simulink model "Leg_4DOF_HGO_v1"  (R2017a)
settings: Solver=VariableStepAuto  StartTime=0.0  StopTime=10  MaxStep=1e-2  RelTol=1e-3  EnableMultiTasking=on
values from neighbouring files (symbols this model uses):
  Amp = [ 1 ; pi/2*ones(3,1) ]    [Copy_of_Init_4DOF.m]
  Ar = [zeros(4) eye(4); zeros(4) zeros(4)]    [Copy_of_Init_HGO_v2.m]    (also in Init_HGO.m; Init_HGO_v1.m; Init_HGO_zoh_v2.m)
  beta = 10    [Copy_of_Init_4DOF.m]
  BodyContact = [ 4 4 ]    [Copy_of_Init_4DOF.m]
  BodyContactPositions = [ contact_point_h, contact_point_t ]    [Copy_of_Init_4DOF.m]
  Br = [zeros(4); eye(4)]    [Copy_of_Init_HGO_v2.m]    (also in Init_HGO.m; Init_HGO_v1.m; Init_HGO_zoh_v2.m)
  Cr = [eye(4) zeros(4)]    [Copy_of_Init_HGO_v2.m]    (also in Init_HGO.m; Init_HGO_v1.m; Init_HGO_zoh_v2.m)
  dqInit = [ 0 0 0 0 ]'    [Copy_of_Init_4DOF.m]
  G = g*ez    [Copy_of_Init_4DOF.m]
  G_ctrl = g*ez    [Copy_of_Init_4DOF.m]
  h = [ ez -ey -ey -ey ]    [Copy_of_Init_4DOF.m]
  h_ctrl = [ ez -ey -ey -ey ]    [Copy_of_Init_4DOF.m]
  Hmu = [eye(4)/Mu zeros(4); zeros(4) eye(4)/Mu^2]    [Copy_of_Init_HGO_v2.m]    (also in Init_HGO.m; Init_HGO_v1.m; Init_HGO_zoh_v2.m)
  Inertia = [ I_base I_hip I_thigh I_shin I_foot ]    [Copy_of_Init_4DOF.m]
  Inertia_ctrl = [ I_base I_hip I_thigh I_shin I_foot ]    [Copy_of_Init_4DOF.m]
  joint_type = [ 1 0 0 0 ]    [Copy_of_Init_4DOF.m]
  k_b = 10    [Copy_of_Init_4DOF.m]
  Kd = kd*eye(n)    [Copy_of_Init_4DOF.m]
  Ki = ki*eye(n)    [Copy_of_Init_4DOF.m]
  Kp = kp*eye(n)    [Copy_of_Init_4DOF.m]
  L = [ l_base_hip l_hip_thigh l_thigh_shin l_shin_foot ]    [Copy_of_Init_4DOF.m]
  L_ctrl = [ l_base_hip l_hip_thigh l_thigh_shin l_shin_foot ]    [Copy_of_Init_4DOF.m]
  L_hgo = [2*eye(4);6*eye(4)]    [Copy_of_Init_HGO_v2.m]    (also in Init_HGO.m = [eye(4);2*eye(4)]; Init_HGO_v1.m = [eye(4);2*eye(4)]; Init_HGO_zoh_v2.m)
  Mass = [ mass_base mass_hip mass_thigh mass_shin mass_foot ]    [Copy_of_Init_4DOF.m]
  Mass_ctrl = [ mass_base mass_hip mass_thigh mass_shin mass_foot ]    [Copy_of_Init_4DOF.m]
  offset = zeros(n,1)    [Copy_of_Init_4DOF.m]
  qInit = [ 0 pi/2 -pi/2 0 ]'    [Copy_of_Init_4DOF.m]
  R = [ r_base r_hip r_thigh r_shin r_foot ]    [Copy_of_Init_4DOF.m]
  R_ctrl = [ r_base r_hip r_thigh r_shin r_foot ]    [Copy_of_Init_4DOF.m]
  s_z = 2    [Copy_of_Init_4DOF.m]
  w = [ 0   ; 0.5*pi*ones(3,1) ]    [Copy_of_Init_4DOF.m]
undefined symbols (not defined in the file or in its folder): Fstate0
settings Model: Creator=Ultron  LastModifiedBy=ignacio
settings DataIOCC: LimitDataPoints=on  SaveFormat=Array
settings OptimizationCC: LifeSpan=inf
settings DebuggingCC: SFUnexpectedBacktrackingDiag=warning  SFNoUnconditionalDefaultTransitionDiag=warning  SFExecutionAtInitializationDiag=none
settings HardwareCC: ProdBitPerPointer=32  ProdBitPerSizeT=32  ProdBitPerPtrDiffT=32  ProdLargestAtomicFloat=None  ProdIntDivRoundTo=Undefined  ProdEndianess=Unspecified  ProdWordSize=32  ProdHWDeviceType=32-bit Generic
settings ModelReferenceCC: PropagateSignalLabelsOutOfModel=off
settings GRTTargetCC: TargetLangStandard=C89/C90 (ANSI)  GeneratePreprocessorConditionals=Disable all
settings ConfigComp: CovMetricSettings=dw  CovHtmlReporting=on  CovSaveCumulativeToWorkspaceVar=on  CovSaveSingleToWorkspaceVar=on  CovExternalEMLEnable=off

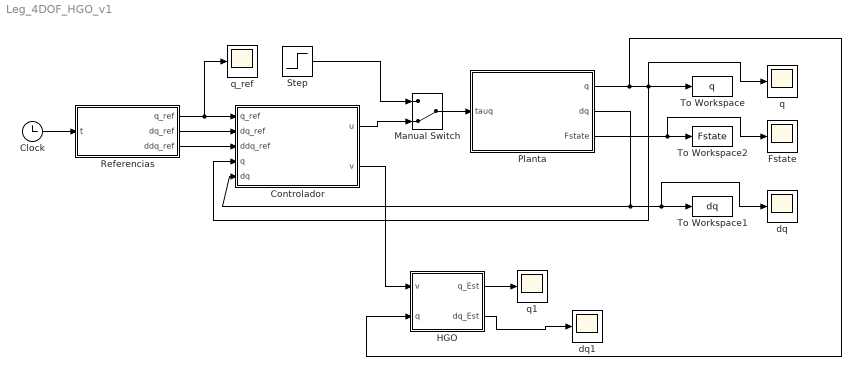
== system Leg_4DOF_HGO_v1 ==
  Clock : Clock
  Controlador : Subsystem
  Fstate : Scope
  HGO : Subsystem
  Manual Switch : ManualSwitch  CurrentSetting=0
  Planta : Subsystem
  Referencias : MATLAB Function  TreatAsAtomicUnit=on
  Step : Step  Before=[0;0;0;0]  After=[0;0;0;0]  SampleTime=0
  To Workspace : ToWorkspace  VariableName=q  SaveFormat=Timeseries  SampleTime=-1
  To Workspace1 : ToWorkspace  VariableName=dq  SaveFormat=Timeseries  SampleTime=-1
  To Workspace2 : ToWorkspace  VariableName=Fstate  SaveFormat=Timeseries  SampleTime=-1
  dq : Scope
  dq1 : Scope
  q : Scope
  q1 : Scope
  q_ref : Scope
  wires:
  Planta/2(dq) -> dq/1, To Workspace1/1, Controlador/5(dq)
  Manual Switch/1 -> Planta/1(tauq)
  Step/1 -> Manual Switch/1
  Controlador/1(u) -> Manual Switch/2
  Referencias/1(q_ref) -> q_ref/1, Controlador/1(q_ref)
  Referencias/2(dq_ref) -> Controlador/2(dq_ref)
  Referencias/3(ddq_ref) -> Controlador/3(ddq_ref)
  Clock/1 -> Referencias/1(t)
  Planta/1(q) -> HGO/2(q), Controlador/4(q), To Workspace/1, q/1
  Planta/3(Fstate) -> Fstate/1, To Workspace2/1
  HGO/1(q_Est) -> q1/1
  HGO/2(dq_Est) -> dq1/1
  Controlador/2(v) -> HGO/1(v)

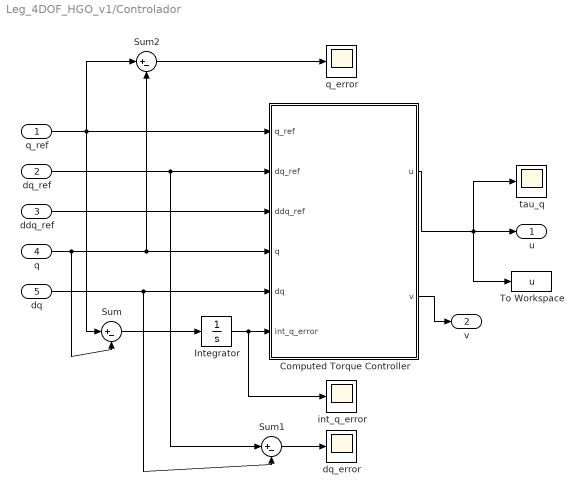
== system Leg_4DOF_HGO_v1/Controlador ==
  q_ref : Inport
  dq_ref : Inport  Port=2
  ddq_ref : Inport  Port=3
  q : Inport  Port=4
  dq : Inport  Port=5
  Computed Torque Controller : MATLAB Function  TreatAsAtomicUnit=on
  Integrator : Integrator  InitialCondition=zeros(4,1)
  Sum : Sum  Inputs=|+-
  Sum1 : Sum  Inputs=|+-
  Sum2 : Sum  Inputs=|+-
  To Workspace : ToWorkspace  VariableName=u  SaveFormat=Timeseries  SampleTime=-1
  dq_error : Scope
  int_q_error : Scope
  q_error : Scope
  tau_q : Scope
  u : Outport
  v : Outport  Port=2
  wires:
  Computed Torque Controller/1(u) -> To Workspace/1, tau_q/1, u/1
  q_ref/1 -> Sum2/1, Sum/1, Computed Torque Controller/1(q_ref)
  dq_ref/1 -> Sum1/1, Computed Torque Controller/2(dq_ref)
  q/1 -> Sum/2, Computed Torque Controller/4(q), Sum2/2
  Sum1/1 -> dq_error/1
  ddq_ref/1 -> Computed Torque Controller/3(ddq_ref)
  dq/1 -> Sum1/2, Computed Torque Controller/5(dq)
  Sum/1 -> Integrator/1
  Integrator/1 -> int_q_error/1, Computed Torque Controller/6(int_q_error)
  Sum2/1 -> q_error/1
  Computed Torque Controller/2(v) -> v/1

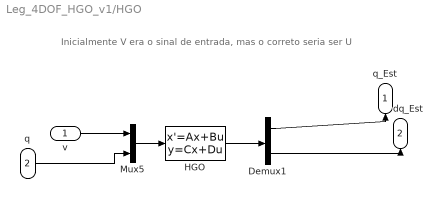
== system Leg_4DOF_HGO_v1/HGO ==
  note: Inicialmente V era o sinal de entrada, mas o correto seria ser U
  v : Inport
  q : Inport  Port=2
  Demux1 : Demux  Outputs=2
  HGO : StateSpace  A=Ar-Hmu*L_hgo*Cr  B=[Br Hmu*L_hgo]  C=eye(8)  D=zeros(8)  X0=[0.01;0.01;0.01;0.01;0.04;0.04;0.04;0.04]
  Mux5 : Mux  Inputs=2
  q_Est : Outport
  dq_Est : Outport  Port=2
  wires:
  Mux5/1 -> HGO/1
  Demux1/1 -> q_Est/1
  Demux1/2 -> dq_Est/1
  v/1 -> Mux5/1
  q/1 -> Mux5/2
  HGO/1 -> Demux1/1

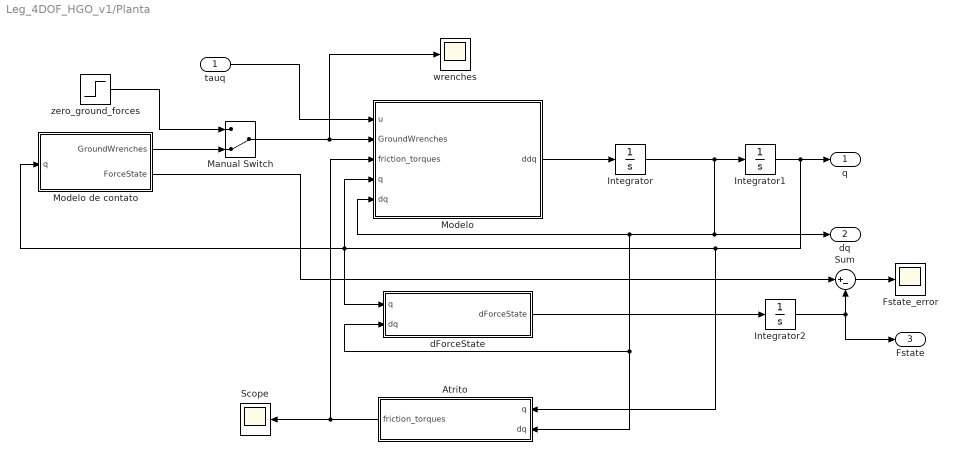
== system Leg_4DOF_HGO_v1/Planta ==
  tauq : Inport
  Atrito : MATLAB Function  TreatAsAtomicUnit=on
  Fstate_error : Scope
  Integrator : Integrator  InitialCondition=dqInit
  Integrator1 : Integrator  InitialCondition=qInit
  Integrator2 : Integrator  InitialCondition=Fstate0
  Manual Switch : ManualSwitch  CurrentSetting=0
  Modelo : MATLAB Function  TreatAsAtomicUnit=on
  Modelo de contato : MATLAB Function  TreatAsAtomicUnit=on
  Scope : Scope
  Sum : Sum  Inputs=|+-
  dForceState : MATLAB Function  TreatAsAtomicUnit=on
  wrenches : Scope
  zero_ground_forces : Step  Before=zeros(6,2)  After=zeros(6,2)  SampleTime=0
  q : Outport
  dq : Outport  Port=2
  Fstate : Outport  Port=3
  wires:
  Integrator1/1 -> dForceState/1(q), Modelo de contato/1(q), Modelo/4(q), Atrito/1(q), q/1
  Integrator/1 -> Integrator1/1, Modelo/5(dq), dForceState/2(dq), Atrito/2(dq), dq/1
  Atrito/1(friction_torques) -> Modelo/3(friction_torques), Scope/1
  tauq/1 -> Modelo/1(u)
  Integrator2/1 -> Sum/2, Fstate/1
  dForceState/1(dForceState) -> Integrator2/1
  Modelo de contato/2(ForceState) -> Sum/1
  Sum/1 -> Fstate_error/1
  Manual Switch/1 -> wrenches/1, Modelo/2(GroundWrenches)
  Modelo de contato/1(GroundWrenches) -> Manual Switch/2
  zero_ground_forces/1 -> Manual Switch/1
  Modelo/1(ddq) -> Integrator/1

== matlab function Leg_4DOF_HGO_v1/Controlador/Computed Torque Controller ==
  data: q_ref input; dq_ref input; ddq_ref input; u output; q input; dq input; int_q_error input; joint_type parameter; Mass_ctrl parameter; Inertia_ctrl parameter; R_ctrl parameter; L_ctrl parameter; h_ctrl parameter; G_ctrl parameter; Kp parameter; Kd parameter; Ki parameter; v output
function [u,v] = fcn(q_ref, dq_ref, ddq_ref, q, dq, int_q_error, joint_type, Mass_ctrl, Inertia_ctrl, R_ctrl, L_ctrl, h_ctrl, G_ctrl, Kp, Kd, Ki )
%% Prostectics control

v = ddq_ref + Kd*(dq_ref - dq) + Kp*(q_ref - q) + Ki*int_q_error;
u = prosthetics_inverse_dynamics( q, dq, v, joint_type, Mass_ctrl, Inertia_ctrl, R_ctrl, L_ctrl, h_ctrl, G_ctrl );

== matlab function Leg_4DOF_HGO_v1/Planta/Modelo ==
  data: u input; GroundWrenches input; friction_torques input; q input; dq input; joint_type parameter; Mass parameter; Inertia parameter; R parameter; L parameter; h parameter; G parameter; ddq output; BodyContactPositions parameter; BodyContact parameter
function ddq = fcn( u, GroundWrenches, friction_torques, q, dq, joint_type, Mass, Inertia, R, L, h, G, BodyContactPositions,  BodyContact )
% direct dynamics

% n = length(q);

% coder.extrinsic('model_prosthetics_mex');
% ddq = coder.nullcopy(zeros(n,1));
% Friction_torques = coder.nullcopy(zeros(n,1));

ddq = model_prosthetics( u, q, dq, joint_type, Mass, Inertia, R, L, h, G, friction_torques, BodyContact, GroundWrenches, BodyContactPositions );
% ddq = model_prosthetics_mex( u, q, dq, joint_type, Mass, Inertia, R, L, h, G, friction_coefs, BodyContact, BodyContactWrenches, BodyContactPositions );

== matlab function Leg_4DOF_HGO_v1/Referencias ==
  data: t input; q_ref output; dq_ref output; ddq_ref output; Amp parameter; offset parameter; w parameter
function [ q_ref, dq_ref, ddq_ref ] = fcn( t, Amp, offset, w)
% generate reference

% q_ref = A*sin(w*t + offset);
% dq_ref = A*w*cos(w*t + offset);
% ddq_ref = -A*(w^2)*sin(w*t + offset);

q_ref = zeros(4,1);
dq_ref = zeros(4,1);
ddq_ref = zeros(4,1);

for i = 1:4
    q_ref(i) = Amp(i)*sin(w(i)*t + offset(i));
    dq_ref(i) = Amp(i)*w(i)*cos(w(i)*t + offset(i));
    ddq_ref(i) = -Amp(i)*(w(i)^2)*sin(w(i)*t + offset(i));
end

== matlab function Leg_4DOF_HGO_v1/Planta/Atrito ==
  data: friction_torques output; q input; dq input
function friction_torques = fcn( q, dq )
%% Joint friction model
n = length(q);
friction_torques = zeros(n,1);

== matlab function Leg_4DOF_HGO_v1/Planta/Modelo de contato ==
  data: GroundWrenches output; q input; BodyContactPositions parameter; s_z parameter; L parameter; h parameter; beta parameter; k_b parameter; joint_type parameter; ForceState output
function [ GroundWrenches, ForceState ] = fcn( q, BodyContactPositions, s_z, L, h, beta,  k_b, joint_type )
% function BodyContactWrenches = fcn( t, q, L, h, BodyContactPositions, joint_type, sz, beta, kb)
% Esta função calcula as forças de contato com o chão

[ GroundWrenches, ForceState ] = ground_model( q, BodyContactPositions, s_z, L, h, beta,  k_b, joint_type );

== matlab function Leg_4DOF_HGO_v1/Planta/dForceState ==
  data: q input; dq input; dForceState output; L parameter; h parameter; joint_type parameter; BodyContactPositions parameter; s_z parameter; beta parameter; k_b parameter
function dForceState = fcn( q, dq, L, h, joint_type,  BodyContactPositions, s_z, beta, k_b)
%% Dinâmica do modelo de contato (em coordenadas inerciais)

%% Computes the velocity body twist of the given point.
body = 4;
contact_point_h = BodyContactPositions(:,1);
contact_point_t = BodyContactPositions(:,2);
V_h = prosthetics_diff_kinematics( q, dq, L, h, body, contact_point_h, joint_type );
V_t = prosthetics_diff_kinematics( q, dq, L, h, body, contact_point_t, joint_type );

%% Computes 
[ P_h, R_h ] = prosthetics_forward_kinematics( q, L, h, body, contact_point_h, joint_type );
[ P_t, R_t ] = prosthetics_forward_kinematics( q, L, h, body, contact_point_h, joint_type );
z_h = P_h(3);
z_t = P_t(3);

%% Converts body linear velocity into inertial velocty
v_h = R_h*V_h(1:3);
v_t = R_t*V_t(1:3);

dz_h = v_h(3);
dz_t = v_t(3);

dF_zh = -(k_b/2)*dz_h*(1+sign(z_h - s_z));
dF_zt = -(k_b/2)*dz_t*(1+sign(z_t - s_z));

dF_xh = beta*dF_zh;
dF_xt = beta*dF_zt;

dForceState = [ dF_zh dF_zt dF_xh dF_xt ]';
